simulink model "convertidor_inversor_2"  (R2020b)
settings: Solver=VariableStepAuto  StartTime=0.0  StopTime=0.4  RelTol=1e-3
InitFcn:
  | Ts = 100e-6;
StartFcn:
  | Ts = 100e-6;
undefined symbols (not defined in the file): Ion, Lithium
libraries: powerlib x38, powerlib_meascontrol x11, slpidlib x10, electricdrivelib x1, simulink x1
(part 2 of 2)

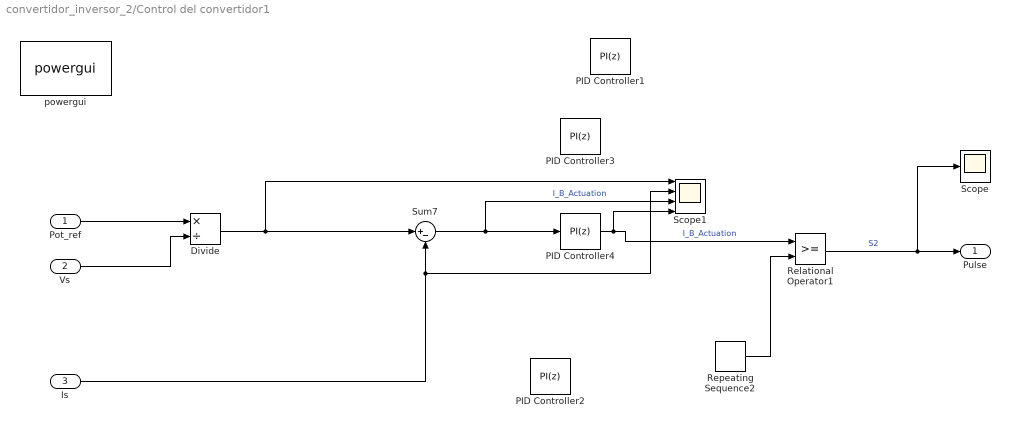
== system convertidor_inversor_2/Control del convertidor1 ==
  Pot_ref : Inport
  Vs : Inport  Port=2
  Is : Inport  Port=3
  Divide : Product  Inputs=*/
  PID Controller1 : slpidlib/PID Controller  Controller=PI  Form=Parallel  TimeDomain=Discrete-time  UseExternalTs=off  SampleTime=Ts  IntegratorMethod=Forward Euler  FilterMethod=Forward Euler  ControllerParametersSource=internal  P=0.01  I=0.02  D=0  UseFilter=on  N=100  TunerSelectOption=Transfer Function Based (PID Tuner App)  InitialConditionSource=internal  InitialConditionForIntegrator=0  InitialConditionForFilter=0  DifferentiatorICPrevScaledInput=0  ExternalReset=none  TrackingMode=off  Kt=1  LimitOutput=on  SatLimitsSource=internal  UpperSaturationLimit=0.95  LowerSaturationLimit=0  LinearizeAsGain=on  AntiWindupMode=clamping  Kb=1  POutMin=[]  POutMax=[]  IOutMin=[]  IOutMax=[]  DOutMin=[]  DOutMax=[]  NOutMin=[]  NOutMax=[]  SumOutMin=[]  SumOutMax=[]  SaturationOutMin=[]  SaturationOutMax=[]  PParamMin=[]  PParamMax=[]  IParamMin=[]  IParamMax=[]  DParamMin=[]  DParamMax=[]  NParamMin=[]  NParamMax=[]  KbParamMin=[]  KbParamMax=[]  KtParamMin=[]  KtParamMax=[]  KbOutMin=[]  KbOutMax=[]  KtOutMin=[]  KtOutMax=[]  IntegratorOutMin=[]  IntegratorOutMax=[]  FilterOutMin=[]  FilterOutMax=[]  SumI1OutMin=[]  SumI1OutMax=[]  SumI2OutMin=[]  SumI2OutMax=[]  SumI3OutMin=[]  SumI3OutMax=[]  SumI4OutMin=[]  SumI4OutMax=[]  SumDOutMin=[]  SumDOutMax=[]  DifferentiatorOutMin=[]  DifferentiatorOutMax=[]  FilterDiffOutCoefMin=[]  FilterDiffOutCoefMax=[]  ReciprocalOutMin=[]  ReciprocalOutMax=[]  SumDenOutMin=[]  SumDenOutMax=[]  SumNumOutMin=[]  SumNumOutMax=[]  DivideOutMin=[]  DivideOutMax=[]  UdiffTsProdOutMin=[]  UdiffTsProdOutMax=[]  NTsProdOutMin=[]  NTsProdOutMax=[]  UintegralTsProdOutMin=[]  UintegralTsProdOutMax=[]  UngainTsProdOutMin=[]  UngainTsProdOutMax=[]  IntegratorContinuousStateAttributes=''  IntegratorStateMustResolveToSignalObject=off  IntegratorRTWStateStorageClass=Auto  FilterContinuousStateAttributes=''  FilterStateMustResolveToSignalObject=off  FilterRTWStateStorageClass=Auto  ParallelPVariant=InternalParameters  IdealPVariant=Disabled  IVariant=InternalParameters  DVariant=Disabled  IntegratorVariant=Discrete  SatVariant=Enabled  AWVariant=DiscClampingParallel  PCopyVariant=Disabled  TRVariant=Disabled  FdbkBlocksVariant=Forward  IdealPFdbkVariant=Disabled  SatFdbkVariant=Disabled  DerivativeFilterVariant=Disabled  NVariant=Disabled  NCopyVariant=Disabled_SignalSpec  FilterICVariant=Disabled  IntegratorICVariant=InternalICs  ExternalResetVariant=Disabled  TRSumVariant=Passthrough  SumFdbkVariant=Disabled  SumVariant=Sum_PI  TsampFilterVariant=InternalTs  TsampNgainVariant=Passthrough  TsampIntegralVariant=Passthrough  ExternalSaturationOutDataTypeStr=Inherit: Same as second input
  PID Controller2 : slpidlib/PID Controller  Controller=PI  Form=Parallel  TimeDomain=Discrete-time  UseExternalTs=off  SampleTime=Ts  IntegratorMethod=Forward Euler  FilterMethod=Forward Euler  ControllerParametersSource=internal  P=0.009  I=0  D=0  UseFilter=on  N=100  TunerSelectOption=Transfer Function Based (PID Tuner App)  InitialConditionSource=internal  InitialConditionForIntegrator=0  InitialConditionForFilter=0  DifferentiatorICPrevScaledInput=0  ExternalReset=none  TrackingMode=off  Kt=1  LimitOutput=on  SatLimitsSource=internal  UpperSaturationLimit=0.95  LowerSaturationLimit=0  LinearizeAsGain=on  AntiWindupMode=clamping  Kb=1  POutMin=[]  POutMax=[]  IOutMin=[]  IOutMax=[]  DOutMin=[]  DOutMax=[]  NOutMin=[]  NOutMax=[]  SumOutMin=[]  SumOutMax=[]  SaturationOutMin=[]  SaturationOutMax=[]  PParamMin=[]  PParamMax=[]  IParamMin=[]  IParamMax=[]  DParamMin=[]  DParamMax=[]  NParamMin=[]  NParamMax=[]  KbParamMin=[]  KbParamMax=[]  KtParamMin=[]  KtParamMax=[]  KbOutMin=[]  KbOutMax=[]  KtOutMin=[]  KtOutMax=[]  IntegratorOutMin=[]  IntegratorOutMax=[]  FilterOutMin=[]  FilterOutMax=[]  SumI1OutMin=[]  SumI1OutMax=[]  SumI2OutMin=[]  SumI2OutMax=[]  SumI3OutMin=[]  SumI3OutMax=[]  SumI4OutMin=[]  SumI4OutMax=[]  SumDOutMin=[]  SumDOutMax=[]  DifferentiatorOutMin=[]  DifferentiatorOutMax=[]  FilterDiffOutCoefMin=[]  FilterDiffOutCoefMax=[]  ReciprocalOutMin=[]  ReciprocalOutMax=[]  SumDenOutMin=[]  SumDenOutMax=[]  SumNumOutMin=[]  SumNumOutMax=[]  DivideOutMin=[]  DivideOutMax=[]  UdiffTsProdOutMin=[]  UdiffTsProdOutMax=[]  NTsProdOutMin=[]  NTsProdOutMax=[]  UintegralTsProdOutMin=[]  UintegralTsProdOutMax=[]  UngainTsProdOutMin=[]  UngainTsProdOutMax=[]  IntegratorContinuousStateAttributes=''  IntegratorStateMustResolveToSignalObject=off  IntegratorRTWStateStorageClass=Auto  FilterContinuousStateAttributes=''  FilterStateMustResolveToSignalObject=off  FilterRTWStateStorageClass=Auto  ParallelPVariant=InternalParameters  IdealPVariant=Disabled  IVariant=InternalParameters  DVariant=Disabled  IntegratorVariant=Discrete  SatVariant=Enabled  AWVariant=DiscClampingParallel  PCopyVariant=Disabled  TRVariant=Disabled  FdbkBlocksVariant=Forward  IdealPFdbkVariant=Disabled  SatFdbkVariant=Disabled  DerivativeFilterVariant=Disabled  NVariant=Disabled  NCopyVariant=Disabled_SignalSpec  FilterICVariant=Disabled  IntegratorICVariant=InternalICs  ExternalResetVariant=Disabled  TRSumVariant=Passthrough  SumFdbkVariant=Disabled  SumVariant=Sum_PI  TsampFilterVariant=InternalTs  TsampNgainVariant=Passthrough  TsampIntegralVariant=Passthrough  ExternalSaturationOutDataTypeStr=Inherit: Same as second input
  PID Controller3 : slpidlib/PID Controller  Controller=PI  Form=Parallel  TimeDomain=Discrete-time  UseExternalTs=off  SampleTime=Ts  IntegratorMethod=Forward Euler  FilterMethod=Forward Euler  ControllerParametersSource=internal  P=0.001  I=0.02  D=0  UseFilter=on  N=100  TunerSelectOption=Transfer Function Based (PID Tuner App)  InitialConditionSource=internal  InitialConditionForIntegrator=0  InitialConditionForFilter=0  DifferentiatorICPrevScaledInput=0  ExternalReset=none  TrackingMode=off  Kt=1  LimitOutput=on  SatLimitsSource=internal  UpperSaturationLimit=0.95  LowerSaturationLimit=0  LinearizeAsGain=on  AntiWindupMode=clamping  Kb=1  POutMin=[]  POutMax=[]  IOutMin=[]  IOutMax=[]  DOutMin=[]  DOutMax=[]  NOutMin=[]  NOutMax=[]  SumOutMin=[]  SumOutMax=[]  SaturationOutMin=[]  SaturationOutMax=[]  PParamMin=[]  PParamMax=[]  IParamMin=[]  IParamMax=[]  DParamMin=[]  DParamMax=[]  NParamMin=[]  NParamMax=[]  KbParamMin=[]  KbParamMax=[]  KtParamMin=[]  KtParamMax=[]  KbOutMin=[]  KbOutMax=[]  KtOutMin=[]  KtOutMax=[]  IntegratorOutMin=[]  IntegratorOutMax=[]  FilterOutMin=[]  FilterOutMax=[]  SumI1OutMin=[]  SumI1OutMax=[]  SumI2OutMin=[]  SumI2OutMax=[]  SumI3OutMin=[]  SumI3OutMax=[]  SumI4OutMin=[]  SumI4OutMax=[]  SumDOutMin=[]  SumDOutMax=[]  DifferentiatorOutMin=[]  DifferentiatorOutMax=[]  FilterDiffOutCoefMin=[]  FilterDiffOutCoefMax=[]  ReciprocalOutMin=[]  ReciprocalOutMax=[]  SumDenOutMin=[]  SumDenOutMax=[]  SumNumOutMin=[]  SumNumOutMax=[]  DivideOutMin=[]  DivideOutMax=[]  UdiffTsProdOutMin=[]  UdiffTsProdOutMax=[]  NTsProdOutMin=[]  NTsProdOutMax=[]  UintegralTsProdOutMin=[]  UintegralTsProdOutMax=[]  UngainTsProdOutMin=[]  UngainTsProdOutMax=[]  IntegratorContinuousStateAttributes=''  IntegratorStateMustResolveToSignalObject=off  IntegratorRTWStateStorageClass=Auto  FilterContinuousStateAttributes=''  FilterStateMustResolveToSignalObject=off  FilterRTWStateStorageClass=Auto  ParallelPVariant=InternalParameters  IdealPVariant=Disabled  IVariant=InternalParameters  DVariant=Disabled  IntegratorVariant=Discrete  SatVariant=Enabled  AWVariant=DiscClampingParallel  PCopyVariant=Disabled  TRVariant=Disabled  FdbkBlocksVariant=Forward  IdealPFdbkVariant=Disabled  SatFdbkVariant=Disabled  DerivativeFilterVariant=Disabled  NVariant=Disabled  NCopyVariant=Disabled_SignalSpec  FilterICVariant=Disabled  IntegratorICVariant=InternalICs  ExternalResetVariant=Disabled  TRSumVariant=Passthrough  SumFdbkVariant=Disabled  SumVariant=Sum_PI  TsampFilterVariant=InternalTs  TsampNgainVariant=Passthrough  TsampIntegralVariant=Passthrough  ExternalSaturationOutDataTypeStr=Inherit: Same as second input
  PID Controller4 : slpidlib/PID Controller  Controller=PI  Form=Parallel  TimeDomain=Discrete-time  UseExternalTs=off  SampleTime=Ts  IntegratorMethod=Forward Euler  FilterMethod=Forward Euler  ControllerParametersSource=internal  P=0.06  I=0  D=0  UseFilter=on  N=100  TunerSelectOption=Transfer Function Based (PID Tuner App)  InitialConditionSource=internal  InitialConditionForIntegrator=0  InitialConditionForFilter=0  DifferentiatorICPrevScaledInput=0  ExternalReset=none  TrackingMode=off  Kt=1  LimitOutput=on  SatLimitsSource=internal  UpperSaturationLimit=0.95  LowerSaturationLimit=0  LinearizeAsGain=on  AntiWindupMode=clamping  Kb=1  POutMin=[]  POutMax=[]  IOutMin=[]  IOutMax=[]  DOutMin=[]  DOutMax=[]  NOutMin=[]  NOutMax=[]  SumOutMin=[]  SumOutMax=[]  SaturationOutMin=[]  SaturationOutMax=[]  PParamMin=[]  PParamMax=[]  IParamMin=[]  IParamMax=[]  DParamMin=[]  DParamMax=[]  NParamMin=[]  NParamMax=[]  KbParamMin=[]  KbParamMax=[]  KtParamMin=[]  KtParamMax=[]  KbOutMin=[]  KbOutMax=[]  KtOutMin=[]  KtOutMax=[]  IntegratorOutMin=[]  IntegratorOutMax=[]  FilterOutMin=[]  FilterOutMax=[]  SumI1OutMin=[]  SumI1OutMax=[]  SumI2OutMin=[]  SumI2OutMax=[]  SumI3OutMin=[]  SumI3OutMax=[]  SumI4OutMin=[]  SumI4OutMax=[]  SumDOutMin=[]  SumDOutMax=[]  DifferentiatorOutMin=[]  DifferentiatorOutMax=[]  FilterDiffOutCoefMin=[]  FilterDiffOutCoefMax=[]  ReciprocalOutMin=[]  ReciprocalOutMax=[]  SumDenOutMin=[]  SumDenOutMax=[]  SumNumOutMin=[]  SumNumOutMax=[]  DivideOutMin=[]  DivideOutMax=[]  UdiffTsProdOutMin=[]  UdiffTsProdOutMax=[]  NTsProdOutMin=[]  NTsProdOutMax=[]  UintegralTsProdOutMin=[]  UintegralTsProdOutMax=[]  UngainTsProdOutMin=[]  UngainTsProdOutMax=[]  IntegratorContinuousStateAttributes=''  IntegratorStateMustResolveToSignalObject=off  IntegratorRTWStateStorageClass=Auto  FilterContinuousStateAttributes=''  FilterStateMustResolveToSignalObject=off  FilterRTWStateStorageClass=Auto  ParallelPVariant=InternalParameters  IdealPVariant=Disabled  IVariant=InternalParameters  DVariant=Disabled  IntegratorVariant=Discrete  SatVariant=Enabled  AWVariant=DiscClampingParallel  PCopyVariant=Disabled  TRVariant=Disabled  FdbkBlocksVariant=Forward  IdealPFdbkVariant=Disabled  SatFdbkVariant=Disabled  DerivativeFilterVariant=Disabled  NVariant=Disabled  NCopyVariant=Disabled_SignalSpec  FilterICVariant=Disabled  IntegratorICVariant=InternalICs  ExternalResetVariant=Disabled  TRSumVariant=Passthrough  SumFdbkVariant=Disabled  SumVariant=Sum_PI  TsampFilterVariant=InternalTs  TsampNgainVariant=Passthrough  TsampIntegralVariant=Passthrough  ExternalSaturationOutDataTypeStr=Inherit: Same as second input
  Relational Operator1 : RelationalOperator  OutDataTypeStr=boolean  RndMeth=Nearest
  Repeating Sequence2 : simulink/Sources/Repeating Sequence  rep_seq_t=[0 Ts/2 Ts]  rep_seq_y=[0 1 0]
  Scope : Scope
  Scope1 : Scope  NumInputPorts=4
  Sum7 : Sum  Inputs=|+-
  powergui : powerlib/powergui  Priority=1  SimulationMode=Discrete  SampleTime=1e-5  frequency=60  Iterations=50  frequencyindice=0  Pbase=100e6  ErrMax=1e-4  UnitsV=kV  UnitsW=MW  buscounter=0  FunctionMessages=off  echomessages=off  EnableUseOfTLC=off  CurrentSourceSwitches=off  DisableSnubberDevices=off  DisableRonSwitches=off  DisableVfSwitches=off  DisplayEquations=off  AutomaticDiscreteSolvers=off  SolverType=Tustin/Backward Euler (TBE)  Interpol=off  ExternalGateDelay=off  methode=off  Ts=100  x0status=blocks  SPID=on  SwTol=0  HookPort=off  NonlinearTolerance=1e-4  nMaxIteration=100  ContinueOnMaxIteration=off  RestoreLinks=warning  ResistiveCurrentMeasurement=off  Frange=[0:2:500]  Ylog=off  Xlog=on  ShowGrid=off  save=off  variable=ZData  structure=0  ZoomFFT=off  StartTime=0.0  cycles=1  DisplayStyle=1  fundamental=60  FreqAxis=off  MaxFrequency=1000  frequencyindicesteady=1  RmsSteady=1  display=off
  Pulse : Outport
  wires:
  Vs/1 -> Divide/2
  Divide/1 -> Sum7/1, Scope1/1
  PID Controller4/1 -> Relational Operator1/1, Scope1/4  "I_B_Actuation"
  Sum7/1 -> Scope1/3, PID Controller4/1  "I_B_Actuation"
  Relational Operator1/1 -> Pulse/1, Scope/1  "S2"
  Repeating Sequence2/1 -> Relational Operator1/2
  Pot_ref/1 -> Divide/1
  Is/1 -> Sum7/2, Scope1/2

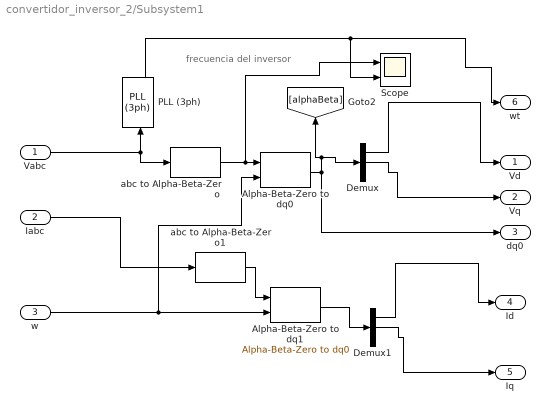
== system convertidor_inversor_2/Subsystem1 ==
  note: frecuencia del inversor
  Vabc : Inport
  Iabc : Inport  Port=2
  w : Inport  Port=3
  Alpha-Beta-Zero to dq0 : powerlib_meascontrol/Transformations/Alpha-Beta-Zero to dq0  Alignment=90 degrees behind phase A axis
  Alpha-Beta-Zero to dq1 : powerlib_meascontrol/Transformations/Alpha-Beta-Zero to dq0  Alignment=90 degrees behind phase A axis
  Demux : Demux  Outputs=3
  Demux1 : Demux  Outputs=3
  PLL (3ph) : powerlib_meascontrol/PLL/PLL (3ph)  Fmin=45  Par_Init=[0, 50]  ParK=[180, 3200, 1]  TcD=1e-4  MaxRateChangeFreq=12  FilterCutOffFreq=25  Ts=0  AGC=on
  Scope : Scope  NumInputPorts=2
  abc to Alpha-Beta-Zero : powerlib_meascontrol/Transformations/abc to Alpha-Beta-Zero
  abc to Alpha-Beta-Zero1 : powerlib_meascontrol/Transformations/abc to Alpha-Beta-Zero
  Vd : Outport
  Vq : Outport  Port=2
  dq0 : Outport  Port=3
  Id : Outport  Port=4
  Iq : Outport  Port=5
  wt : Outport  Port=6
  wires:
  PLL (3ph)/2 -> Scope/2, wt/1
  Iabc/1 -> abc to Alpha-Beta-Zero1/1
  Demux/1 -> Vd/1
  w/1 -> Alpha-Beta-Zero to dq1/2, Alpha-Beta-Zero to dq0/2
  Vabc/1 -> abc to Alpha-Beta-Zero/1, PLL (3ph)/1
  Alpha-Beta-Zero to dq1/1 -> Demux1/1
  abc to Alpha-Beta-Zero1/1 -> Alpha-Beta-Zero to dq1/1
  abc to Alpha-Beta-Zero/1 -> Alpha-Beta-Zero to dq0/1, Scope/1
  Alpha-Beta-Zero to dq0/1 -> [alphaBeta], Demux/1, dq0/1
  Demux1/2 -> Iq/1
  Demux1/1 -> Id/1
  Demux/2 -> Vq/1

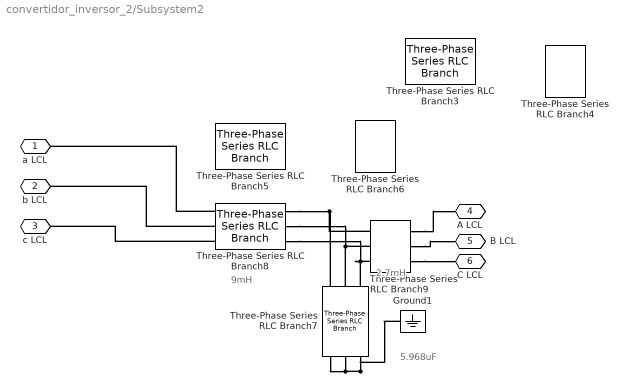
== system convertidor_inversor_2/Subsystem2 ==
  note: 2.7mH
  note: 9mH
  note: 5.968uF
  Ground1 : powerlib/Elements/Ground  LConnTagsString=a
  Three-Phase Series RLC Branch3 : powerlib/Elements/Three-Phase Series RLC Branch  LConnTagsString=A|B|C  RConnTagsString=A|B|C  BranchType=L  Resistance=1  Inductance=3.186e-3  Capacitance=1e-6  Measurements=None
  Three-Phase Series RLC Branch4 : powerlib/Elements/Three-Phase Series RLC Branch  LConnTagsString=A|B|C  RConnTagsString=A|B|C  BranchType=L  Resistance=1  Inductance=1.186e-3  Capacitance=1e-6  Measurements=None
  Three-Phase Series RLC Branch5 : powerlib/Elements/Three-Phase Series RLC Branch  LConnTagsString=A|B|C  RConnTagsString=A|B|C  BranchType=L  Resistance=1  Inductance=4.186e-3  Capacitance=1e-6  Measurements=None
  Three-Phase Series RLC Branch6 : powerlib/Elements/Three-Phase Series RLC Branch  LConnTagsString=A|B|C  RConnTagsString=A|B|C  BranchType=L  Resistance=1  Inductance=1.186e-3  Capacitance=1e-6  Measurements=None
  Three-Phase Series RLC Branch7 : powerlib/Elements/Three-Phase Series RLC Branch  LConnTagsString=A|B|C  RConnTagsString=A|B|C  BranchType=C  Resistance=1  Inductance=1e-3  Capacitance=1.8236e-5  Measurements=None
  Three-Phase Series RLC Branch8 : powerlib/Elements/Three-Phase Series RLC Branch  LConnTagsString=A|B|C  RConnTagsString=A|B|C  BranchType=L  Resistance=1  Inductance=5.586e-3  Capacitance=1e-6  Measurements=None
  Three-Phase Series RLC Branch9 : powerlib/Elements/Three-Phase Series RLC Branch  LConnTagsString=A|B|C  RConnTagsString=A|B|C  BranchType=L  Resistance=1  Inductance=0.100e-3  Capacitance=1e-6  Measurements=None
  a LCL : PMIOPort  Side=Right
  "b LCL " : PMIOPort  Port=2  Side=Right
  c LCL : PMIOPort  Port=3  Side=Right
  A LCL : PMIOPort  Port=4  Side=Left
  B LCL : PMIOPort  Port=5  Side=Left
  C LCL : PMIOPort  Port=6  Side=Left
  connections:
  Three-Phase Series RLC Branch9/LConn3 -- C LCL/RConn1
  Three-Phase Series RLC Branch9/LConn1 -- A LCL/RConn1
  Three-Phase Series RLC Branch9/LConn2 -- B LCL/RConn1
  Three-Phase Series RLC Branch8/RConn2 -- "b LCL "/RConn1
  Three-Phase Series RLC Branch8/RConn1 -- a LCL/RConn1
  Three-Phase Series RLC Branch8/LConn3 -- Three-Phase Series RLC Branch7/LConn3 -- Three-Phase Series RLC Branch9/RConn3
  Three-Phase Series RLC Branch8/RConn3 -- c LCL/RConn1
  Three-Phase Series RLC Branch8/LConn2 -- Three-Phase Series RLC Branch7/LConn2 -- Three-Phase Series RLC Branch9/RConn2
  Three-Phase Series RLC Branch8/LConn1 -- Three-Phase Series RLC Branch7/LConn1 -- Three-Phase Series RLC Branch9/RConn1
  Ground1/LConn1 -- Three-Phase Series RLC Branch7/RConn3 -- Three-Phase Series RLC Branch7/RConn1 -- Three-Phase Series RLC Branch7/RConn2

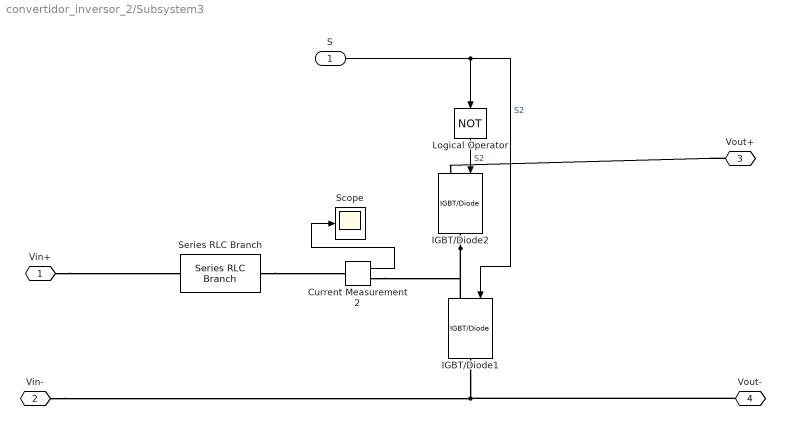
== system convertidor_inversor_2/Subsystem3 ==
  S : Inport
  Current Measurement2 : powerlib/Measurements/Current Measurement  PhasorSimulation=off  OutputType=Complex  PSBequivalent=0
  IGBT/Diode1 : powerlib/Power Electronics/IGBT//Diode  Ron=1e-3  Rs=1e5  Cs=inf  Measurements=off
  IGBT/Diode2 : powerlib/Power Electronics/IGBT//Diode  Ron=1e-3  Rs=1e5  Cs=inf  Measurements=off
  Logical Operator : Logic  Operator=NOT  AllPortsSameDT=off  OutDataTypeStr=boolean
  Scope : Scope
  Series RLC Branch : powerlib/Elements/Series RLC Branch  LConnTagsString=__new0  RConnTagsString=__new0  BranchType=L  Resistance=3  Inductance=30e-3  SetiL0=off  InitialCurrent=0  Capacitance=1e-6  Setx0=off  InitialVoltage=0  Measurements=None
  Vin+ : PMIOPort  Side=Left
  Vin- : PMIOPort  Port=2  Side=Left
  Vout+ : PMIOPort  Port=3  Side=Right
  Vout- : PMIOPort  Port=4  Side=Right
  wires:
  Current Measurement2/1 -> Scope/1
  Logical Operator/1 -> IGBT/Diode2/1  "S2"
  S/1 -> Logical Operator/1, IGBT/Diode1/1  "S2"
  connections:
  Vout+/RConn1 -- IGBT/Diode2/LConn1
  IGBT/Diode2/RConn1 -- Current Measurement2/RConn1 -- IGBT/Diode1/LConn1
  Vin+/RConn1 -- Series RLC Branch/LConn1
  Series RLC Branch/RConn1 -- Current Measurement2/LConn1
  IGBT/Diode1/RConn1 -- Vout-/RConn1 -- Vin-/RConn1

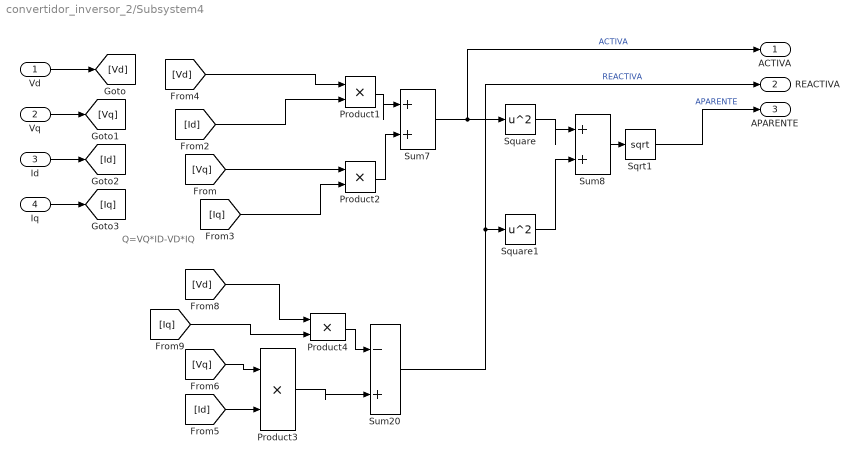
== system convertidor_inversor_2/Subsystem4 ==
  note: Q=VQ*ID-VD*IQ
  Vd : Inport
  Vq : Inport  Port=2
  Id : Inport  Port=3
  Iq : Inport  Port=4
  Product{1..4} (4 alike) : Product
  Sqrt1 : Sqrt  SaturateOnIntegerOverflow=on
  Square : Math  Operator=square  SaturateOnIntegerOverflow=on
  Square1 : Math  Operator=square  SaturateOnIntegerOverflow=on
  Sum20 : Sum  Inputs=|-+
  Sum7 : Sum  Inputs=|++
  Sum8 : Sum  Inputs=|++
  ACTIVA : Outport
  REACTIVA : Outport  Port=2
  APARENTE : Outport  Port=3
  wires:
  [Iq] -> Product4/2
  Vd/1 -> [Vd]
  Vq/1 -> [Vq]
  Id/1 -> [Id]
  Iq/1 -> [Iq]
  [Id] -> Product1/2
  [Id] -> Product3/2
  Product3/1 -> Sum20/2
  [Vq] -> Product3/1
  [Vd] -> Product4/1
  Product4/1 -> Sum20/1
  Square1/1 -> Sum8/2
  Sum20/1 -> Square1/1, REACTIVA/1  "REACTIVA"
  Sqrt1/1 -> APARENTE/1  "APARENTE"
  [Vd] -> Product1/1
  [Vq] -> Product2/1
  [Iq] -> Product2/2
  Sum8/1 -> Sqrt1/1
  Sum7/1 -> Square/1, ACTIVA/1  "ACTIVA"
  Square/1 -> Sum8/1
  Product2/1 -> Sum7/2
  Product1/1 -> Sum7/1

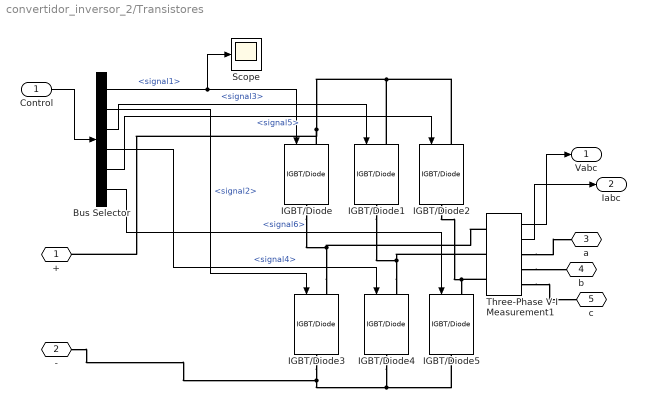
== system convertidor_inversor_2/Transistores ==
  Control : Inport
  Bus Selector : BusSelector  OutputSignals=signal1,signal2,signal3,signal4,signal5,signal6
  IGBT/Diode{,1..5} (6 alike) : powerlib/Power Electronics/IGBT//Diode  Ron=1e-3  Rs=1e5  Cs=inf  Measurements=off
  Scope : Scope
  Three-Phase V-I Measurement1 : powerlib/Measurements/Three-Phase V-I Measurement  VoltageMeasurement=phase-to-phase  SetLabelV=off  LabelV=Vabc  Vpu=off  VpuLL=off  CurrentMeasurement=yes  SetLabelI=off  LabelI=Iabc  Ipu=off  Pbase=100e6  Vbase=500e3  OutputType=Complex  PhasorSimulation=off  PSBequivalent=0
  + : PMIOPort  Side=Left
  - : PMIOPort  Port=2  Side=Left
  a : PMIOPort  Port=3  Side=Right
  b : PMIOPort  Port=4  Side=Right
  c : PMIOPort  Port=5  Side=Right
  Vabc : Outport
  Iabc : Outport  Port=2
  wires:
  Bus Selector/6 -> IGBT/Diode5/1  "<signal6>"
  Bus Selector/5 -> IGBT/Diode2/1  "<signal5>"
  Bus Selector/4 -> IGBT/Diode4/1  "<signal4>"
  Bus Selector/3 -> IGBT/Diode1/1  "<signal3>"
  Bus Selector/2 -> IGBT/Diode3/1  "<signal2>"
  Control/1 -> Bus Selector/1
  Bus Selector/1 -> Scope/1, IGBT/Diode/1  "<signal1>"
  Three-Phase V-I Measurement1/1 -> Vabc/1
  Three-Phase V-I Measurement1/2 -> Iabc/1
  connections:
  Three-Phase V-I Measurement1/RConn2 -- b/RConn1
  Three-Phase V-I Measurement1/RConn1 -- a/RConn1
  Three-Phase V-I Measurement1/RConn3 -- c/RConn1
  IGBT/Diode5/RConn1 -- IGBT/Diode4/RConn1 -- -/RConn1 -- IGBT/Diode3/RConn1
  +/RConn1 -- IGBT/Diode/LConn1 -- IGBT/Diode2/LConn1 -- IGBT/Diode1/LConn1
  IGBT/Diode5/LConn1 -- Three-Phase V-I Measurement1/LConn3 -- IGBT/Diode2/RConn1
  IGBT/Diode4/LConn1 -- Three-Phase V-I Measurement1/LConn2 -- IGBT/Diode1/RConn1
  IGBT/Diode3/LConn1 -- Three-Phase V-I Measurement1/LConn1 -- IGBT/Diode/RConn1

== matlab function convertidor_inversor_2/MATLAB Function ==
  data: IN input; Current output; Enable output
%BLOQUE YA HECHO CON EL REPARTO 28/09/2023

function [Current,Enable]    = Ctr_V(IN)

 persistent val;
 
 if isempty(val)
     val=0;
 end
  
if IN >= 600
    Current =80;
    Enable= true;
    val=1;
elseif IN < 600 && val==1
    Current =80;
    Enable= true;
else
   Current=0;
   Enable=false;
end
    
 
% 
% function [Current,Enable]    = P_REG(IN)
% 
% persistent dato;
% 
% if isempty(dato)
%     dato=0;
%     
% end
%         
% if IN >= 550
%    dato=dato+10;
%    if dato>=50
%      Current = 80;
%      Enable=true;
%    else
%       Current=0;
%       Enable=false;
%    end      
% else
%    Current=0;
%    Enable=false;
% end
%
